simulink model "pidControlled"  (R2018b)
settings: Solver=VariableStepAuto  StartTime=0.0  StopTime=t_stop  RelTol=1e-3
values from neighbouring files (symbols this model uses):
  b_1 = 5e2    (= 500)    [mechatronicsProject2019_Group29.m]
  b_2 = 5e2    (= 500)    [mechatronicsProject2019_Group29.m]
  b_motor = 5e-3    (= 0.005)    [mechatronicsProject2019_Group29.m]
  c = 2*P_cut/(w_c^3)    (= 8.6712271875e-05)    [mechatronicsProject2019_Group29.m]
  d_PID = 0    [mechatronicsProject2019_Group29.m]
  i_PID = 0    [mechatronicsProject2019_Group29.m]
  J_c = (pi*rho_c*t*D_c^4)/(32)    (= 0.0930760146353)    [mechatronicsProject2019_Group29.m]
  J_m = 0.0064    [mechatronicsProject2019_Group29.m]
  k = (G_steel*pi*d_shaft^4)/(32*l_shaft)    (= 11626.0526632)    [mechatronicsProject2019_Group29.m]
  K_e = 0.149    [mechatronicsProject2019_Group29.m]
  K_t = T_rated/i_a    (= 2.4)    [mechatronicsProject2019_Group29.m]
  K_tach = 0.0289    [mechatronicsProject2019_Group29.m]
  L_a = 6.6e-3    (= 0.0066)    [mechatronicsProject2019_Group29.m]
  p_PID = 1.6018878881e11    (= 160188788810)    [mechatronicsProject2019_Group29.m]
  R_a = 0.65    [mechatronicsProject2019_Group29.m]
  t_cut_start = 5    [mechatronicsProject2019_Group29.m]
  t_cut_stop = 1.5*t_cut_start    (= 7.5)    [mechatronicsProject2019_Group29.m]
  t_step = 0    [mechatronicsProject2019_Group29.m]
  w_c = 2*V_c/D_c    (= 444.444444444)    [mechatronicsProject2019_Group29.m]
libraries: simulink x2
settings Model: Creator=tumisang  LastModifiedBy=tumisang

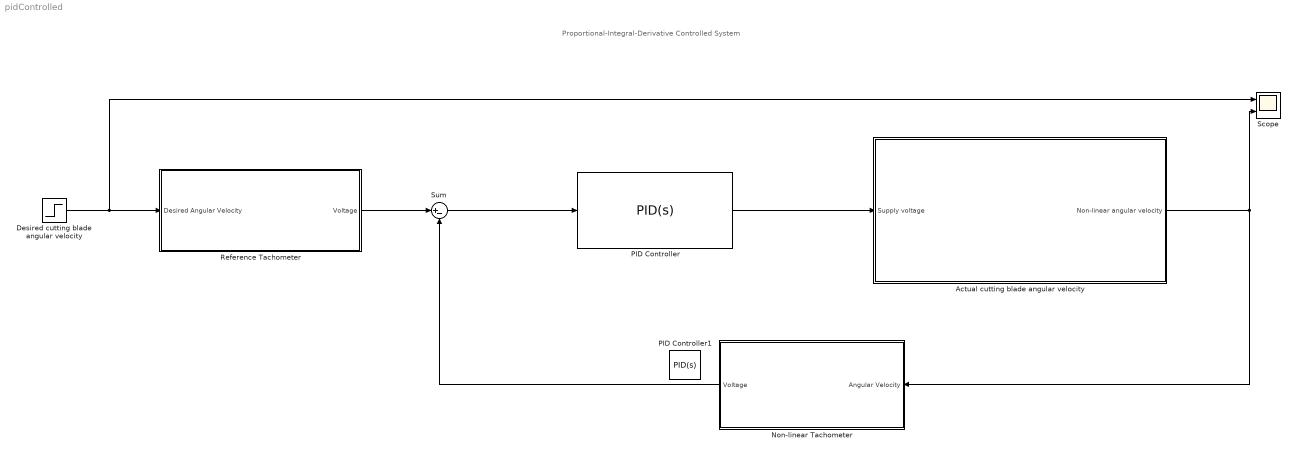
== system pidControlled ==
  note: Proportional-Integral-Derivative Controlled System
  Actual cutting blade angular velocity : Subsystem
  Desired cutting blade angular velocity : Step  Time=t_step  After=w_c  SampleTime=0
  Non-linear Tachometer : Subsystem
  PID Controller : simulink/Continuous/PID Controller  Controller=PID  Form=Ideal  TimeDomain=Continuous-time  SampleTime=-1  IntegratorMethod=Forward Euler  FilterMethod=Forward Euler  ControllerParametersSource=internal  P=p_PID  I=i_PID  D=d_PID  UseFilter=on  N=100  TunerSelectOption=Transfer Function Based (PID Tuner App)  InitialConditionSource=internal  InitialConditionForIntegrator=0  InitialConditionForFilter=0  DifferentiatorICPrevScaledInput=0  ExternalReset=none  TrackingMode=off  Kt=1  LimitOutput=off  UpperSaturationLimit=inf  LowerSaturationLimit=-inf  LinearizeAsGain=on  AntiWindupMode=none  Kb=1  POutMin=[]  POutMax=[]  IOutMin=[]  IOutMax=[]  DOutMin=[]  DOutMax=[]  NOutMin=[]  NOutMax=[]  SumOutMin=[]  SumOutMax=[]  SaturationOutMin=[]  SaturationOutMax=[]  PParamMin=[]  PParamMax=[]  IParamMin=[]  IParamMax=[]  DParamMin=[]  DParamMax=[]  NParamMin=[]  NParamMax=[]  KbParamMin=[]  KbParamMax=[]  KtParamMin=[]  KtParamMax=[]  KbOutMin=[]  KbOutMax=[]  KtOutMin=[]  KtOutMax=[]  IntegratorOutMin=[]  IntegratorOutMax=[]  FilterOutMin=[]  FilterOutMax=[]  SumI1OutMin=[]  SumI1OutMax=[]  SumI2OutMin=[]  SumI2OutMax=[]  SumI3OutMin=[]  SumI3OutMax=[]  SumI4OutMin=[]  SumI4OutMax=[]  SumDOutMin=[]  SumDOutMax=[]  DifferentiatorOutMin=[]  DifferentiatorOutMax=[]  FilterDiffOutCoefMin=[]  FilterDiffOutCoefMax=[]  ReciprocalOutMin=[]  ReciprocalOutMax=[]  SumDenOutMin=[]  SumDenOutMax=[]  SumNumOutMin=[]  SumNumOutMax=[]  DivideOutMin=[]  DivideOutMax=[]  IntegratorContinuousStateAttributes=''  IntegratorStateMustResolveToSignalObject=off  IntegratorRTWStateStorageClass=Auto  FilterContinuousStateAttributes=''  FilterStateMustResolveToSignalObject=off  FilterRTWStateStorageClass=Auto  ParallelPVariant=Passthrough  IdealPVariant=InternalParameters  IVariant=InternalParameters  DVariant=InternalParameters  IntegratorVariant=Continuous  SatVariant=Disabled  AWVariant=Passthrough  PCopyVariant=Disabled  TRVariant=Disabled  FdbkBlocksVariant=Forward  IdealPFdbkVariant=Disabled  SatFdbkVariant=Disabled  DerivativeFilterVariant=ContFilter  NVariant=InternalParameters  NCopyVariant=Disabled  FilterICVariant=InternalICsFilter  IntegratorICVariant=InternalICs  ExternalResetVariant=Disabled  TRSumVariant=Passthrough  SumFdbkVariant=Disabled  SumVariant=Sum_PID
  PID Controller1 : simulink/Continuous/PID Controller  Controller=PID  Form=Parallel  TimeDomain=Continuous-time  SampleTime=-1  IntegratorMethod=Forward Euler  FilterMethod=Forward Euler  ControllerParametersSource=internal  P=1  I=1  D=0  UseFilter=on  N=100  TunerSelectOption=Transfer Function Based (PID Tuner App)  InitialConditionSource=internal  InitialConditionForIntegrator=0  InitialConditionForFilter=0  DifferentiatorICPrevScaledInput=0  ExternalReset=none  TrackingMode=off  Kt=1  LimitOutput=off  UpperSaturationLimit=inf  LowerSaturationLimit=-inf  LinearizeAsGain=on  AntiWindupMode=none  Kb=1  POutMin=[]  POutMax=[]  IOutMin=[]  IOutMax=[]  DOutMin=[]  DOutMax=[]  NOutMin=[]  NOutMax=[]  SumOutMin=[]  SumOutMax=[]  SaturationOutMin=[]  SaturationOutMax=[]  PParamMin=[]  PParamMax=[]  IParamMin=[]  IParamMax=[]  DParamMin=[]  DParamMax=[]  NParamMin=[]  NParamMax=[]  KbParamMin=[]  KbParamMax=[]  KtParamMin=[]  KtParamMax=[]  KbOutMin=[]  KbOutMax=[]  KtOutMin=[]  KtOutMax=[]  IntegratorOutMin=[]  IntegratorOutMax=[]  FilterOutMin=[]  FilterOutMax=[]  SumI1OutMin=[]  SumI1OutMax=[]  SumI2OutMin=[]  SumI2OutMax=[]  SumI3OutMin=[]  SumI3OutMax=[]  SumI4OutMin=[]  SumI4OutMax=[]  SumDOutMin=[]  SumDOutMax=[]  DifferentiatorOutMin=[]  DifferentiatorOutMax=[]  FilterDiffOutCoefMin=[]  FilterDiffOutCoefMax=[]  ReciprocalOutMin=[]  ReciprocalOutMax=[]  SumDenOutMin=[]  SumDenOutMax=[]  SumNumOutMin=[]  SumNumOutMax=[]  DivideOutMin=[]  DivideOutMax=[]  IntegratorContinuousStateAttributes=''  IntegratorStateMustResolveToSignalObject=off  IntegratorRTWStateStorageClass=Auto  FilterContinuousStateAttributes=''  FilterStateMustResolveToSignalObject=off  FilterRTWStateStorageClass=Auto  ParallelPVariant=InternalParameters  IdealPVariant=Disabled  IVariant=InternalParameters  DVariant=InternalParameters  IntegratorVariant=Continuous  SatVariant=Disabled  AWVariant=Passthrough  PCopyVariant=Disabled  TRVariant=Disabled  FdbkBlocksVariant=Forward  IdealPFdbkVariant=Disabled  SatFdbkVariant=Disabled  DerivativeFilterVariant=ContFilter  NVariant=InternalParameters  NCopyVariant=Disabled  FilterICVariant=InternalICsFilter  IntegratorICVariant=InternalICs  ExternalResetVariant=Disabled  TRSumVariant=Passthrough  SumFdbkVariant=Disabled  SumVariant=Sum_PID
  Reference Tachometer : Subsystem
  Scope : Scope  NumInputPorts=2
  Sum : Sum  Inputs=|+-
  wires:
  Actual cutting blade angular velocity/1("Non-linear angular velocity ") -> Scope/2, Non-linear Tachometer/1(Angular Velocity)
  Non-linear Tachometer/1(Voltage) -> Sum/2
  Reference Tachometer/1(Voltage) -> Sum/1
  Desired cutting blade angular velocity/1 -> Scope/1, Reference Tachometer/1(Desired Angular Velocity)
  PID Controller/1 -> Actual cutting blade angular velocity/1(Supply voltage)
  Sum/1 -> PID Controller/1

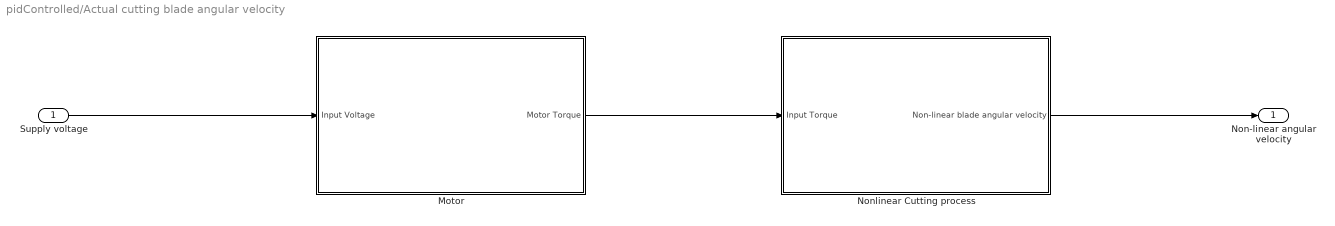
== system pidControlled/Actual cutting blade angular velocity ==
  Supply voltage : Inport
  Motor : Subsystem  Description=Motor
  Nonlinear Cutting process : Subsystem
  "Non-linear angular velocity " : Outport
  wires:
  Motor/1(Motor Torque) -> Nonlinear Cutting process/1(Input Torque)
  Nonlinear Cutting process/1(Non-linear blade angular velocity) -> "Non-linear angular velocity "/1
  Supply voltage/1 -> Motor/1(Input Voltage)

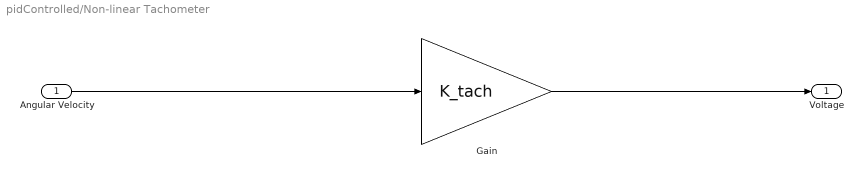
== system pidControlled/Non-linear Tachometer ==
  Angular Velocity : Inport
  Gain : Gain  Gain=K_tach
  Voltage : Outport
  wires:
  Angular Velocity/1 -> Gain/1
  Gain/1 -> Voltage/1

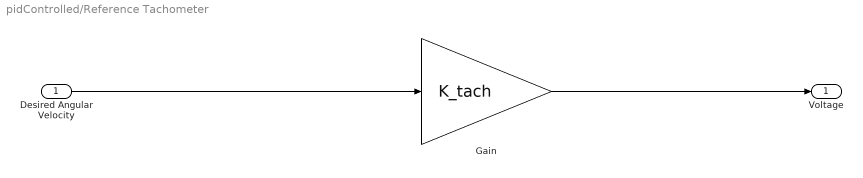
== system pidControlled/Reference Tachometer ==
  Desired Angular Velocity : Inport
  Gain : Gain  Gain=K_tach
  Voltage : Outport
  wires:
  Desired Angular Velocity/1 -> Gain/1
  Gain/1 -> Voltage/1

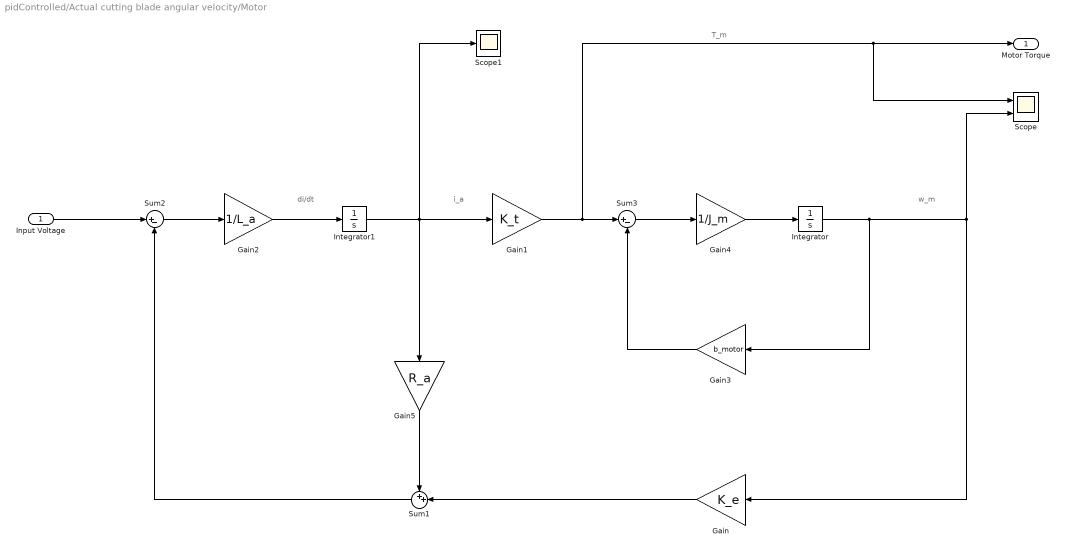
== system pidControlled/Actual cutting blade angular velocity/Motor ==
  note: di/dt
  note: T_m
  note: w_m
  note: i_a
  Input Voltage : Inport
  Gain : Gain  Gain=K_e
  Gain1 : Gain  Gain=K_t
  Gain2 : Gain  Gain=1/L_a
  Gain3 : Gain  Gain=b_motor
  Gain4 : Gain  Gain=1/J_m
  Gain5 : Gain  Gain=R_a
  Integrator : Integrator
  Integrator1 : Integrator
  Scope : Scope  NumInputPorts=2
  Scope1 : Scope
  Sum1 : Sum  Inputs=++|
  Sum2 : Sum  Inputs=|+-
  Sum3 : Sum  Inputs=|+-
  Motor Torque : Outport
  wires:
  Gain/1 -> Sum1/2
  Gain5/1 -> Sum1/1
  Sum1/1 -> Sum2/2
  Sum2/1 -> Gain2/1
  Gain2/1 -> Integrator1/1
  Sum3/1 -> Gain4/1
  Gain4/1 -> Integrator/1
  Integrator/1 -> Gain3/1, Gain/1, Scope/2
  Gain3/1 -> Sum3/2
  Gain1/1 -> Motor Torque/1, Scope/1, Sum3/1
  Input Voltage/1 -> Sum2/1
  Integrator1/1 -> Scope1/1, Gain1/1, Gain5/1

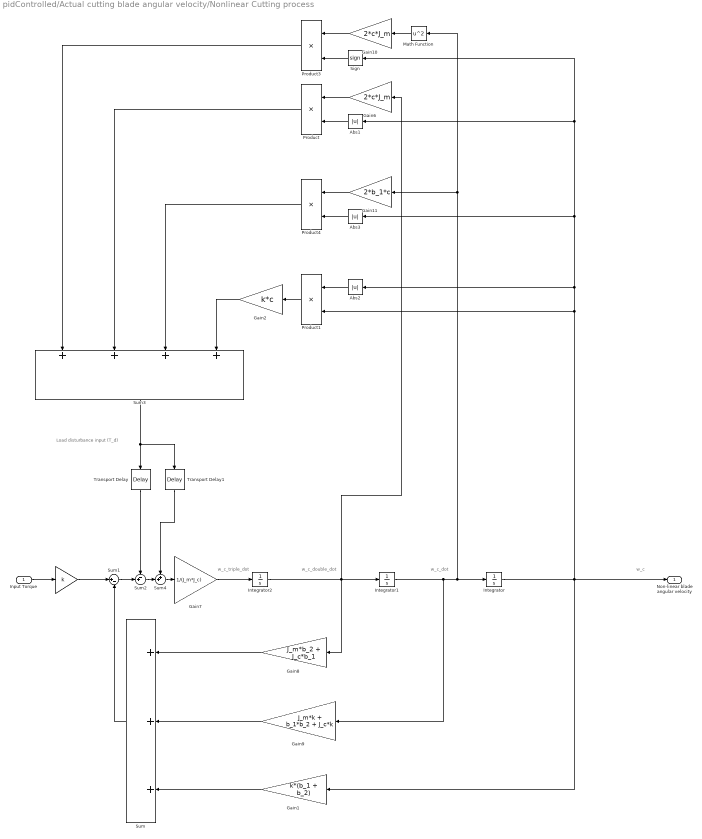
== system pidControlled/Actual cutting blade angular velocity/Nonlinear Cutting process ==
  note: Load disturbance input (T_d)
  note: w_c_dot
  note: w_c
  note: w_c_double_dot
  note: w_c_triple_dot
  Input Torque : Inport
  " " : Gain  Gain=k
  Abs1 : Abs
  Abs2 : Abs
  Abs3 : Abs
  Gain1 : Gain  Gain=k*(b_1 + b_2)
  Gain10 : Gain  Gain=2*c*J_m
  Gain11 : Gain  Gain=2*b_1*c
  Gain2 : Gain  Gain=k*c
  Gain6 : Gain  Gain=2*c*J_m
  Gain7 : Gain  Gain=1/(J_m*J_c)
  Gain8 : Gain  Gain=J_m*b_2 + J_c*b_1
  Gain9 : Gain  Gain=J_m*k + b_1*b_2 + J_c*k
  Integrator : Integrator
  Integrator1 : Integrator
  Integrator2 : Integrator
  Math Function : Math  Operator=square  SaturateOnIntegerOverflow=on
  Product{,1,3..4} (4 alike) : Product
  Sign : Signum
  Sum : Sum  Inputs=+++
  Sum1 : Sum  Inputs=|+-
  Sum2 : Sum  Inputs=-+|
  Sum3 : Sum  Inputs=++++
  Sum4 : Sum  Inputs=++|
  Transport Delay : TransportDelay  DelayTime=t_cut_start  BufferSize=117760
  Transport Delay1 : TransportDelay  DelayTime=t_cut_stop  BufferSize=76800
  Non-linear blade angular velocity : Outport
  wires:
  Input Torque/1 -> " "/1
  " "/1 -> Sum1/1
  Sum/1 -> Sum1/2
  Gain7/1 -> Integrator2/1
  Integrator2/1 -> Integrator1/1, Gain6/1, Gain8/1
  Integrator/1 -> Abs3/1, Sign/1, Abs1/1, Abs2/1, Product1/2, Non-linear blade angular velocity/1, Gain1/1
  Gain8/1 -> Sum/1
  Gain6/1 -> Product/1
  Abs1/1 -> Product/2
  Gain9/1 -> Sum/2
  Gain10/1 -> Product3/1
  Math Function/1 -> Gain10/1
  Gain11/1 -> Product4/1
  Integrator1/1 -> Gain11/1, Math Function/1, Integrator/1, Gain9/1
  Abs3/1 -> Product4/2
  Sign/1 -> Product3/2
  Product1/1 -> Gain2/1
  Abs2/1 -> Product1/1
  Sum2/1 -> Sum4/2
  Sum1/1 -> Sum2/2
  Product3/1 -> Sum3/1
  Product/1 -> Sum3/2
  Gain1/1 -> Sum/3
  Product4/1 -> Sum3/3
  Gain2/1 -> Sum3/4
  Transport Delay/1 -> Sum2/1
  Sum3/1 -> Transport Delay1/1, Transport Delay/1
  Sum4/1 -> Gain7/1
  Transport Delay1/1 -> Sum4/1
